simulink model "quadruped"  (R2019b)
settings: Solver=ode23t  StartTime=0.0  StopTime=Ts  RelTol=1e-3
values from neighbouring files (symbols this model uses):
  isdone = Isdone    [RL_reward.m]
  plane = [5, 50, 0.03]    [quadruped_sim_param.m]
  reward = Reward    [RL_reward.m]
  robot = Robot    [quadruped_sim_param.m]
undefined symbols (not defined in the file or in its folder): X, Y, Z
libraries: sm_lib x166, nesl_utility x90, simulink x33, rllib x1
(part 1 of 6)
settings Model: Creator=krzysiek  LastModifiedBy=dimazhylko
settings SolverCC: ZeroCrossAlgorithm=Adaptive
settings DebuggingCC: IgnoredZcDiagnostic=none
settings DiagnosticsConfigSet: SimMechanicsRigidlyBoundBlock=none

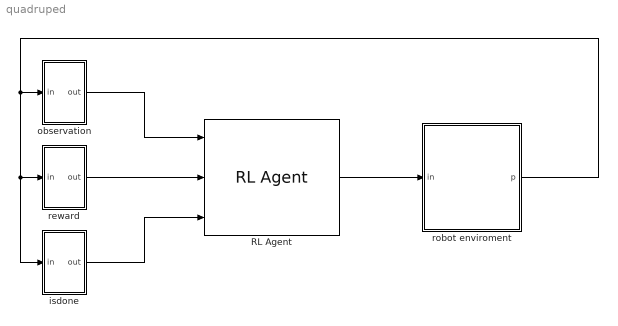
== system quadruped ==
  RL Agent : rllib/RL Agent  Agent=agentObj  ProvideReward=on  ProvideIsDone=on  ProvideCumRwd=off  TreatAsDirectFeedthrough=on  CollectLoggedSignals=on  CollectModelStates=on
      settings: SourceProductName=Reinforcement Learning Toolbox
  isdone : Subsystem  mask{isd=isdone}
  observation : Subsystem
  reward : Subsystem  mask{rew=reward}
  robot enviroment : Subsystem
  wires:
  RL Agent/1 -> robot enviroment/1(in)
  robot enviroment/1(p) -> isdone/1(in), reward/1(in), observation/1(in)
  reward/1(out) -> RL Agent/2
  observation/1(out) -> RL Agent/1
  isdone/1(out) -> RL Agent/3

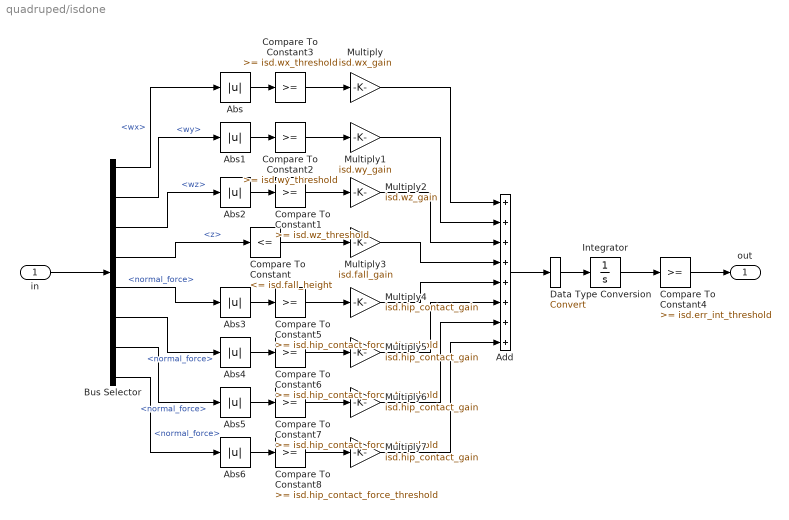
== system quadruped/isdone ==
  in : Inport
  Abs{,1..6} (7 alike) : Abs
  Add : Sum  Inputs=++++++++
  Bus Selector : BusSelector  OutputSignals=body.wx,body.wy,body.wz,body.z,RL.hip.normal_force,FL.hip.normal_force,FR.hip.normal_force,RR.hip.normal_force
  Compare To Constant : simulink/Logic and Bit Operations/Compare To Constant  relop=<=  const=isd.fall_height  OutDataTypeStr=uint8
  Compare To Constant1 : simulink/Logic and Bit Operations/Compare To Constant  relop=>=  const=isd.wz_threshold  OutDataTypeStr=uint8
  Compare To Constant2 : simulink/Logic and Bit Operations/Compare To Constant  relop=>=  const=isd.wy_threshold  OutDataTypeStr=uint8
  Compare To Constant3 : simulink/Logic and Bit Operations/Compare To Constant  relop=>=  const=isd.wx_threshold  OutDataTypeStr=uint8
  Compare To Constant4 : simulink/Logic and Bit Operations/Compare To Constant  relop=>=  const=isd.err_int_threshold  OutDataTypeStr=boolean
  Compare To Constant{5..8} (4 alike) : simulink/Logic and Bit Operations/Compare To Constant  relop=>=  const=isd.hip_contact_force_threshold  OutDataTypeStr=uint8
  Data Type Conversion : DataTypeConversion
  Integrator : Integrator
  Multiply : Gain  Gain=isd.wx_gain
  Multiply1 : Gain  Gain=isd.wy_gain
  Multiply2 : Gain  Gain=isd.wz_gain
  Multiply3 : Gain  Gain=isd.fall_gain
  Multiply{4..7} (4 alike) : Gain  Gain=isd.hip_contact_gain
  out : Outport
  wires:
  in/1 -> Bus Selector/1
  Bus Selector/4 -> Compare To Constant/1  "<z>"
  Abs/1 -> Compare To Constant3/1
  Abs1/1 -> Compare To Constant2/1
  Abs2/1 -> Compare To Constant1/1
  Bus Selector/3 -> Abs2/1  "<wz>"
  Bus Selector/2 -> Abs1/1  "<wy>"
  Bus Selector/1 -> Abs/1  "<wx>"
  Integrator/1 -> Compare To Constant4/1
  Add/1 -> Data Type Conversion/1
  Multiply/1 -> Add/1
  Multiply1/1 -> Add/2
  Multiply2/1 -> Add/3
  Multiply3/1 -> Add/4
  Compare To Constant3/1 -> Multiply/1
  Compare To Constant2/1 -> Multiply1/1
  Compare To Constant1/1 -> Multiply2/1
  Compare To Constant/1 -> Multiply3/1
  Compare To Constant4/1 -> out/1
  Data Type Conversion/1 -> Integrator/1
  Abs3/1 -> Compare To Constant5/1
  Compare To Constant5/1 -> Multiply4/1
  Abs4/1 -> Compare To Constant6/1
  Compare To Constant6/1 -> Multiply5/1
  Abs5/1 -> Compare To Constant7/1
  Compare To Constant7/1 -> Multiply6/1
  Abs6/1 -> Compare To Constant8/1
  Compare To Constant8/1 -> Multiply7/1
  Bus Selector/5 -> Abs3/1  "<normal_force>"
  Bus Selector/6 -> Abs4/1  "<normal_force>"
  Bus Selector/7 -> Abs5/1  "<normal_force>"
  Bus Selector/8 -> Abs6/1  "<normal_force>"
  Multiply5/1 -> Add/6
  Multiply4/1 -> Add/5
  Multiply6/1 -> Add/7
  Multiply7/1 -> Add/8

== system quadruped/observation ==
  in : Inport
  Bus Selector : BusSelector  OutputSignals=RL,FL,FR,RR,body
  Bus Selector{1..4} (4 alike) : BusSelector  OutputSignals=hip.joint.position,leg.lower joint data.position,leg.upper jount data.position,leg.tip.pos,leg.tip.normal_force
  Bus Selector5 : BusSelector  OutputSignals=wx,wy,wz,x,y,z,vx,vy,vz
  Bus Selector{6..9} (4 alike) : BusSelector  OutputSignals=x,y,z
  Mux : Mux  Inputs=37
  out : Outport
  wires:
  in/1 -> Bus Selector/1
  Bus Selector/1 -> Bus Selector1/1  "<RL>"
  Mux/1 -> out/1
  Bus Selector/2 -> Bus Selector2/1  "<FL>"
  Bus Selector/3 -> Bus Selector3/1  "<FR>"
  Bus Selector/4 -> Bus Selector4/1  "<RR>"
  Bus Selector/5 -> Bus Selector5/1  "<body>"
  Bus Selector1/1 -> Mux/1  "<position>"
  Bus Selector1/2 -> Mux/2  "<position>"
  Bus Selector1/3 -> Mux/3  "<position>"
  Bus Selector1/5 -> Mux/7  "<normal_force>"
  Bus Selector2/1 -> Mux/8  "<position>"
  Bus Selector2/2 -> Mux/9  "<position>"
  Bus Selector2/3 -> Mux/10  "<position>"
  Bus Selector2/5 -> Mux/14  "<normal_force>"
  Bus Selector3/1 -> Mux/15  "<position>"
  Bus Selector3/2 -> Mux/16  "<position>"
  Bus Selector3/3 -> Mux/17  "<position>"
  Bus Selector3/5 -> Mux/21  "<normal_force>"
  Bus Selector4/1 -> Mux/22  "<position>"
  Bus Selector4/2 -> Mux/23  "<position>"
  Bus Selector4/3 -> Mux/24  "<position>"
  Bus Selector5/2 -> Mux/30  "<wy>"
  Bus Selector5/3 -> Mux/31  "<wz>"
  Bus Selector5/4 -> Mux/32  "<x>"
  Bus Selector5/5 -> Mux/33  "<y>"
  Bus Selector5/6 -> Mux/34  "<z>"
  Bus Selector5/7 -> Mux/35  "<vx>"
  Bus Selector5/8 -> Mux/36  "<vy>"
  Bus Selector5/9 -> Mux/37  "<vz>"
  Bus Selector2/4 -> Bus Selector6/1  "<pos>"
  Bus Selector6/1 -> Mux/11  "<x>"
  Bus Selector6/2 -> Mux/12  "<y>"
  Bus Selector6/3 -> Mux/13  "<z>"
  Bus Selector1/4 -> Bus Selector7/1  "<pos>"
  Bus Selector7/1 -> Mux/4  "<x>"
  Bus Selector7/2 -> Mux/5  "<y>"
  Bus Selector7/3 -> Mux/6  "<z>"
  Bus Selector4/4 -> Bus Selector8/1  "<pos>"
  Bus Selector8/1 -> Mux/25  "<x>"
  Bus Selector5/1 -> Mux/29  "<wx>"
  Bus Selector8/2 -> Mux/26  "<y>"
  Bus Selector8/3 -> Mux/27  "<z>"
  Bus Selector4/5 -> Mux/28  "<normal_force>"
  Bus Selector3/4 -> Bus Selector9/1  "<pos>"
  Bus Selector9/1 -> Mux/18  "<x>"
  Bus Selector9/2 -> Mux/19  "<y>"
  Bus Selector9/3 -> Mux/20  "<z>"

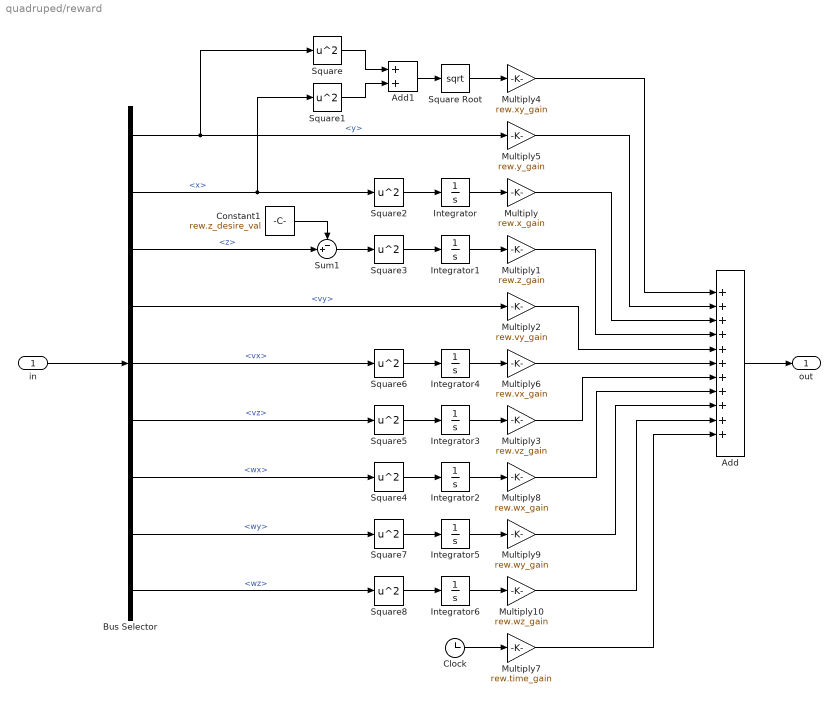
== system quadruped/reward ==
  in : Inport
  Add : Sum  Inputs=+++++++++++
  Add1 : Sum
  Bus Selector : BusSelector  OutputSignals=body.y,body.x,body.z,body.vy,body.vx,body.vz,body.wx,body.wy,body.wz
  Clock : Clock
  Constant1 : Constant  Value=rew.z_desire_val
  Integrator{,1..6} (7 alike) : Integrator
  Multiply : Gain  Gain=rew.x_gain
  Multiply1 : Gain  Gain=rew.z_gain
  Multiply10 : Gain  Gain=rew.wz_gain
  Multiply2 : Gain  Gain=rew.vy_gain
  Multiply3 : Gain  Gain=rew.vz_gain
  Multiply4 : Gain  Gain=rew.xy_gain
  Multiply5 : Gain  Gain=rew.y_gain
  Multiply6 : Gain  Gain=rew.vx_gain
  Multiply7 : Gain  Gain=rew.time_gain
  Multiply8 : Gain  Gain=rew.wx_gain
  Multiply9 : Gain  Gain=rew.wy_gain
  Square : Math  Operator=square  RndMeth=Zero  SaturateOnIntegerOverflow=on
  Square Root : Sqrt  SaturateOnIntegerOverflow=on
  Square1 : Math  Operator=square  RndMeth=Zero  SaturateOnIntegerOverflow=on
  Square{2..8} (7 alike) : Math  Operator=square  SignedPower=off  SaturateOnIntegerOverflow=on
  Sum1 : Sum  Inputs=-+|
  out : Outport
  wires:
  in/1 -> Bus Selector/1
  Square2/1 -> Integrator/1
  Square3/1 -> Integrator1/1
  Sum1/1 -> Square3/1
  Constant1/1 -> Sum1/1
  Square5/1 -> Integrator3/1
  Integrator/1 -> Multiply/1
  Integrator3/1 -> Multiply3/1
  Integrator1/1 -> Multiply1/1
  Add/1 -> out/1
  Add1/1 -> Square Root/1
  Square/1 -> Add1/1
  Square1/1 -> Add1/2
  Square Root/1 -> Multiply4/1
  Multiply4/1 -> Add/1
  Multiply5/1 -> Add/2
  Multiply/1 -> Add/3
  Multiply1/1 -> Add/4
  Multiply6/1 -> Add/6
  Clock/1 -> Multiply7/1
  Multiply3/1 -> Add/7
  Square6/1 -> Integrator4/1
  Integrator4/1 -> Multiply6/1
  Multiply2/1 -> Add/5
  Bus Selector/1 -> Multiply5/1, Square/1  "<y>"
  Bus Selector/2 -> Square2/1, Square1/1  "<x>"
  Bus Selector/3 -> Sum1/2  "<z>"
  Bus Selector/4 -> Multiply2/1  "<vy>"
  Bus Selector/5 -> Square6/1  "<vx>"
  Bus Selector/6 -> Square5/1  "<vz>"
  Square4/1 -> Integrator2/1
  Integrator2/1 -> Multiply8/1
  Square7/1 -> Integrator5/1
  Integrator5/1 -> Multiply9/1
  Square8/1 -> Integrator6/1
  Integrator6/1 -> Multiply10/1
  Bus Selector/7 -> Square4/1  "<wx>"
  Bus Selector/8 -> Square7/1  "<wy>"
  Bus Selector/9 -> Square8/1  "<wz>"
  Multiply8/1 -> Add/8
  Multiply9/1 -> Add/9
  Multiply10/1 -> Add/10
  Multiply7/1 -> Add/11

== system quadruped/robot enviroment ==
  in : Inport
  Bus Creator : BusCreator  Inputs=5
  FL : Subsystem  mask{Leg=robot.RL, plane_dim=plane}
  FR : Subsystem  mask{Leg=robot.FR, plane_dim=plane}
  Mechanism Configuration : sm_lib/Utilities/Mechanism Configuration  UniformGravity=Constant  GravityVector=[0 0 -9.80665]  GravityUnits=m/s^2  LinearizationDelta=0.001
  "Plane " : sm_lib/Body Elements/Brick Solid  GraphicAmbientColor=[0.15 0.15 0.15 1.0]  BasedOnType=Density  BrickDimensions=plane  BrickDimensionUnits=m  CenterOfMass=[0 0 0]  CenterOfMassUnits=m  GraphicDiffuseColor=[0.5 0.5 0.5]  Density=1000  DensityUnits=kg/m^3  DoExposeReferenceFrame=on  GraphicEmissiveColor=[0.0 0.0 0.0 1.0]  ExportEntireGeometry=on  SerializedFrames=<Frames/>  MarkerShape=Sphere  MarkerSize=10  GraphicType=FromGeometry  InertiaType=CalculateFromGeometry  Mass=1  MassUnits=kg  MomentsOfInertia=[1 1 1]  MomentsOfInertiaUnits=kg*m^2  GraphicOpacity=1.0  ProductsOfInertia=[0 0 0]  ProductsOfInertiaUnits=kg*m^2  GraphicShininess=75  GraphicSpecularColor=[0.5 0.5 0.5 1.0]  GraphicVisPropType=SimpleVisualProperties
  RL : Subsystem  mask{Leg=robot.RL, plane_dim=plane}
  RR : Subsystem  mask{Leg=robot.RR, plane_dim=plane}
  Solver Configuration : nesl_utility/Solver Configuration  PhysicalDomain=network_engine_domain  SubClassName=solver  LeftPortType=input  RightPortType=generic  Tones=[]  Harmonics=[]  SimulateNoise=off  Profile=off  UseLocalSampling=off  EnableSwitchedLinearOptims=on  FrequencyDomain=off  UseCCode=off  RelTol=0.001  AbsTol=1e-06  MinStep=1e-09  ToWorkspace=off  RevertToSquareIcSolve=off  NumHomotopyIterations=100  PhasorMode=off  PhasorModeNumHarmonics=1  DoDC=off  ResidualTolerance=1e-09  UseLocalSolver=off  LocalSolverChoice=NE_TRAPEZOIDAL_ADVANCER  LocalSolverSampleTime=0.1  DoFixedCost=off  MaxNonlinIter=3  MaxModeIter=2  LinearAlgebra=Sparse  EquationFormulation=NE_TIME_EF  DelaysMemoryBudget=1024  AutomaticFiltering=on  FilteringTimeConstant=0.001  PartitionStorageMethod=AS_NEEDED  PartitionMemoryBudget=1024  PartitionMethod=FAST
  World Frame : sm_lib/Frames and Transforms/World Frame
  fancy data manipulation : Subsystem
  robot body : Subsystem  mask{robot=robot}
  p : Outport
  wires:
  Bus Creator/1 -> p/1
  robot body/1(p) -> Bus Creator/5  "body"
  RR/1(p) -> Bus Creator/4  "RR"
  FR/1(p) -> Bus Creator/3  "FR"
  FL/1(p) -> Bus Creator/2  "FL"
  RL/1(p) -> Bus Creator/1  "RL"
  in/1 -> fancy data manipulation/1(In1)
  fancy data manipulation/1(Out1) -> RL/1(pos)
  fancy data manipulation/2(Out2) -> FL/1(pos)
  fancy data manipulation/3(Out3) -> RR/1(pos)
  fancy data manipulation/4(Out4) -> FR/1(pos)
  connections:
  RL/RConn2 -- FL/RConn2 -- FR/RConn2 -- RR/RConn2 -- "Plane "/RConn1 -- robot body/LConn2 -- Solver Configuration/RConn1 -- World Frame/RConn1 -- Mechanism Configuration/RConn1
  RR/LConn1 -- robot body/LConn3
  robot body/LConn1 -- RL/LConn1
  FL/LConn1 -- robot body/RConn1
  FR/LConn1 -- robot body/RConn2
  RL/RConn1 -- FL/RConn1 -- FR/RConn1 -- RR/RConn1 -- "Plane "/LConn1

== system quadruped/robot enviroment/FL ==
  pos : Inport
  Bus Creator : BusCreator  Inputs=2
  Constant : Constant  Value=90
  Demux : Demux  Outputs=3
  Multiply : Gain  Gain=180/pi
  Sum : Sum  Inputs=|++
  hip : Subsystem  mask{Hip=Leg.hip}
  leg : Subsystem
  plane : PMIOPort  Side=Right
  B : PMIOPort  Port=2  Side=Left
  F : PMIOPort  Port=3  Side=Right
  p : Outport
  wires:
  Demux/3 -> Multiply/1  "hip pos"
  leg/1(p) -> Bus Creator/2  "leg"
  Bus Creator/1 -> p/1
  pos/1 -> Demux/1
  Demux/1 -> leg/1(up pos)  "leg ang"
  Demux/2 -> leg/2(lo pos)  "knee ang"
  hip/1(p) -> Bus Creator/1  "hip"
  Multiply/1 -> Sum/1
  Sum/1 -> hip/1(pos)
  Constant/1 -> Sum/2
  connections:
  leg/LConn1 -- hip/RConn1
  hip/LConn1 -- B/RConn1
  hip/RConn2 -- plane/RConn1 -- leg/RConn2
  F/RConn1 -- leg/RConn1

== system quadruped/robot enviroment/FR ==
  pos : Inport
  Bus Creator : BusCreator  Inputs=2
  Constant : Constant  Value=90
  Demux : Demux  Outputs=3
  Multiply : Gain  Gain=180/pi
  Sum : Sum  Inputs=|++
  hip : Subsystem  mask{Hip=Leg.hip}
  leg : Subsystem
  plane : PMIOPort  Side=Right
  B : PMIOPort  Port=2  Side=Left
  F : PMIOPort  Port=3  Side=Right
  p : Outport
  wires:
  Demux/3 -> Multiply/1  "hip pos"
  leg/1(p) -> Bus Creator/2  "leg"
  Bus Creator/1 -> p/1
  pos/1 -> Demux/1
  Demux/1 -> leg/1(up pos)  "leg ang"
  Demux/2 -> leg/2(lo pos)  "knee ang"
  hip/1(p) -> Bus Creator/1  "hip"
  Multiply/1 -> Sum/1
  Sum/1 -> hip/1(pos)
  Constant/1 -> Sum/2
  connections:
  leg/LConn1 -- hip/RConn1
  hip/LConn1 -- B/RConn1
  hip/RConn2 -- plane/RConn1 -- leg/RConn2
  F/RConn1 -- leg/RConn1

== system quadruped/robot enviroment/RL ==
  pos : Inport
  Bus Creator : BusCreator  Inputs=2
  Constant : Constant  Value=90
  Demux : Demux  Outputs=3
  Multiply : Gain  Gain=180/pi
  Sum : Sum  Inputs=|++
  hip : Subsystem  mask{Hip=Leg.hip}
  leg : Subsystem
  plane : PMIOPort  Side=Right
  B : PMIOPort  Port=2  Side=Left
  F : PMIOPort  Port=3  Side=Right
  p : Outport
  wires:
  Demux/3 -> Multiply/1  "hip pos"
  leg/1(p) -> Bus Creator/2  "leg"
  Bus Creator/1 -> p/1
  pos/1 -> Demux/1
  Demux/1 -> leg/1(up pos)  "leg ang"
  Demux/2 -> leg/2(lo pos)  "knee ang"
  hip/1(p) -> Bus Creator/1  "hip"
  Multiply/1 -> Sum/1
  Sum/1 -> hip/1(pos)
  Constant/1 -> Sum/2
  connections:
  leg/LConn1 -- hip/RConn1
  hip/LConn1 -- B/RConn1
  hip/RConn2 -- plane/RConn1 -- leg/RConn2
  F/RConn1 -- leg/RConn1

== system quadruped/robot enviroment/RR ==
  pos : Inport
  Bus Creator : BusCreator  Inputs=2
  Constant : Constant  Value=90
  Demux : Demux  Outputs=3
  Multiply : Gain  Gain=180/pi
  Sum : Sum  Inputs=|++
  hip : Subsystem  mask{Hip=Leg.hip}
  leg : Subsystem
  plane : PMIOPort  Side=Right
  B : PMIOPort  Port=2  Side=Left
  F : PMIOPort  Port=3  Side=Right
  p : Outport
  wires:
  Demux/3 -> Multiply/1  "hip pos"
  leg/1(p) -> Bus Creator/2  "leg"
  Bus Creator/1 -> p/1
  pos/1 -> Demux/1
  Demux/1 -> leg/1(up pos)  "leg ang"
  Demux/2 -> leg/2(lo pos)  "knee ang"
  hip/1(p) -> Bus Creator/1  "hip"
  Multiply/1 -> Sum/1
  Sum/1 -> hip/1(pos)
  Constant/1 -> Sum/2
  connections:
  leg/LConn1 -- hip/RConn1
  hip/LConn1 -- B/RConn1
  hip/RConn2 -- plane/RConn1 -- leg/RConn2
  F/RConn1 -- leg/RConn1

== system quadruped/robot enviroment/fancy data manipulation ==
  In1 : Inport
  Demux : Demux  Outputs=12
  Mux{,1..3} (4 alike) : Mux  Inputs=3
  Out1 : Outport
  Out2 : Outport  Port=2
  Out3 : Outport  Port=3
  Out4 : Outport  Port=4
  wires:
  Mux/1 -> Out1/1
  Mux1/1 -> Out2/1
  Mux3/1 -> Out3/1
  In1/1 -> Demux/1
  Mux2/1 -> Out4/1
  Demux/1 -> Mux/1
  Demux/2 -> Mux1/1
  Demux/3 -> Mux2/1
  Demux/4 -> Mux3/1
  Demux/5 -> Mux/2
  Demux/6 -> Mux1/2
  Demux/7 -> Mux2/2
  Demux/8 -> Mux3/2
  Demux/9 -> Mux/3
  Demux/10 -> Mux1/3
  Demux/11 -> Mux2/3
  Demux/12 -> Mux3/3

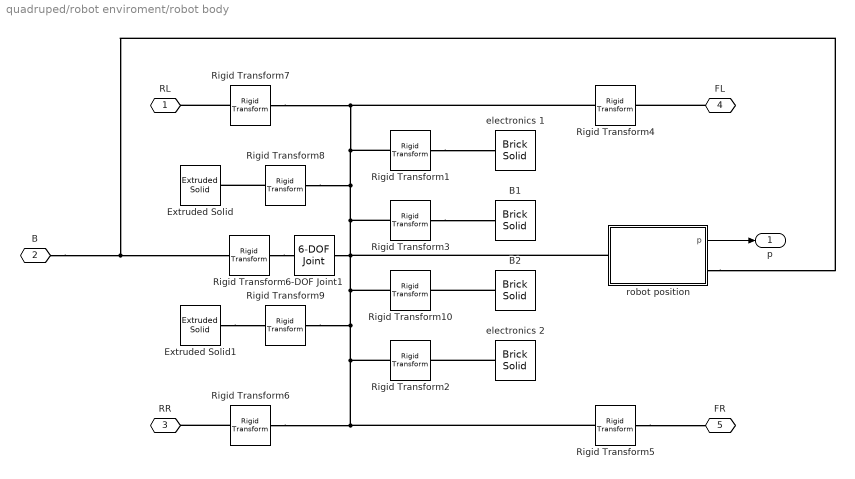
== system quadruped/robot enviroment/robot body ==
  6-DOF Joint1 : sm_lib/Joints/6-DOF Joint  JointMode=Normal  SenseConstraintForce=off  SenseConstraintForceX=off  SenseConstraintForceY=off  SenseConstraintForceZ=off  SenseConstraintTorque=off  SenseConstraintTorqueX=off  SenseConstraintTorqueY=off  SenseConstraintTorqueZ=off  SenseTotalForce=off  SenseTotalForceX=off  SenseTotalForceY=off  SenseTotalForceZ=off  SenseTotalTorque=off  SenseTotalTorqueX=off  SenseTotalTorqueY=off  SenseTotalTorqueZ=off  CompositeWrenchDir=FollowerOnBase  CompositeWrenchFrame=BaseFrame  PxEquilibriumPosition=0  PxEquilibriumPositionUnits=m  PxSpringStiffness=0  PxSpringStiffnessUnits=N/m  PxDampingCoefficient=0  PxDampingCoefficientUnits=N/(m/s)  PxTorqueActuationMode=NoTorque  PxMotionActuationMode=ComputedMotion  PxSensePosition=off  PxSenseVelocity=off  PxSenseAcceleration=off  PxSenseTorqueForce=off  PxSenseLowerLimitTorqueForce=off  PxSenseUpperLimitTorqueForce=off  PxLowerLimitSpecify=off  PxLowerLimitBound=-1  PxLowerLimitBoundUnits=m  PxLowerLimitStiffness=1e6  PxLowerLimitStiffnessUnits=N/m  PxLowerLimitDamping=1e3  PxLowerLimitDampingUnits=N/(m/s)  PxLowerLimitTransitionRegionWidth=1e-4  PxLowerLimitTransitionRegionWidthUnits=m  PxUpperLimitSpecify=off  PxUpperLimitBound=1  PxUpperLimitBoundUnits=m  PxUpperLimitStiffness=1e6  PxUpperLimitStiffnessUnits=N/m  PxUpperLimitDamping=1e3  PxUpperLimitDampingUnits=N/(m/s)  PxUpperLimitTransitionRegionWidth=1e-4  PxUpperLimitTransitionRegionWidthUnits=m  PxPositionTargetSpecify=off  PxPositionTargetPriority=High  PxPositionTargetValue=0  PxPositionTargetValueUnits=m  PxVelocityTargetSpecify=off  PxVelocityTargetPriority=High  PxVelocityTargetValue=0  PxVelocityTargetValueUnits=m/s  PyEquilibriumPosition=0  PyEquilibriumPositionUnits=m  PySpringStiffness=0  PySpringStiffnessUnits=N/m  PyDampingCoefficient=0  PyDampingCoefficientUnits=N/(m/s)  PyTorqueActuationMode=NoTorque  PyMotionActuationMode=ComputedMotion  PySensePosition=off  PySenseVelocity=off  PySenseAcceleration=off  PySenseTorqueForce=off  PySenseLowerLimitTorqueForce=off  PySenseUpperLimitTorqueForce=off  PyLowerLimitSpecify=off  PyLowerLimitBound=-1  PyLowerLimitBoundUnits=m  PyLowerLimitStiffness=1e6  PyLowerLimitStiffnessUnits=N/m  PyLowerLimitDamping=1e3  PyLowerLimitDampingUnits=N/(m/s)  PyLowerLimitTransitionRegionWidth=1e-4  PyLowerLimitTransitionRegionWidthUnits=m  PyUpperLimitSpecify=off  PyUpperLimitBound=1  PyUpperLimitBoundUnits=m  PyUpperLimitStiffness=1e6  PyUpperLimitStiffnessUnits=N/m  PyUpperLimitDamping=1e3  PyUpperLimitDampingUnits=N/(m/s)  PyUpperLimitTransitionRegionWidth=1e-4  PyUpperLimitTransitionRegionWidthUnits=m  PyPositionTargetSpecify=off  PyPositionTargetPriority=High  PyPositionTargetValue=0  PyPositionTargetValueUnits=m  PyVelocityTargetSpecify=off  PyVelocityTargetPriority=High  PyVelocityTargetValue=0  PyVelocityTargetValueUnits=m/s  PzEquilibriumPosition=0  PzEquilibriumPositionUnits=m  PzSpringStiffness=0  PzSpringStiffnessUnits=N/m  PzDampingCoefficient=0  PzDampingCoefficientUnits=N/(m/s)  PzTorqueActuationMode=NoTorque  PzMotionActuationMode=ComputedMotion  PzSensePosition=off  PzSenseVelocity=off  PzSenseAcceleration=off  PzSenseTorqueForce=off  PzSenseLowerLimitTorqueForce=off  PzSenseUpperLimitTorqueForce=off  PzLowerLimitSpecify=off  PzLowerLimitBound=-1  PzLowerLimitBoundUnits=m  PzLowerLimitStiffness=1e6  PzLowerLimitStiffnessUnits=N/m  PzLowerLimitDamping=1e3  PzLowerLimitDampingUnits=N/(m/s)  PzLowerLimitTransitionRegionWidth=1e-4  PzLowerLimitTransitionRegionWidthUnits=m  PzUpperLimitSpecify=off  PzUpperLimitBound=1  PzUpperLimitBoundUnits=m  PzUpperLimitStiffness=1e6  PzUpperLimitStiffnessUnits=N/m  PzUpperLimitDamping=1e3  PzUpperLimitDampingUnits=N/(m/s)  PzUpperLimitTransitionRegionWidth=1e-4  PzUpperLimitTransitionRegionWidthUnits=m  PzPositionTargetSpecify=off  PzPositionTargetPriority=High  PzPositionTargetValue=0  PzPositionTargetValueUnits=m  PzVelocityTargetSpecify=off  PzVelocityTargetPriority=High  PzVelocityTargetValue=0  PzVelocityTargetValueUnits=m/s  SphDefPosRotationMethod=None  SphDefPosRotationAngleUnits=deg  SphDefPosRotationStandardAxis=+Z  SphDefPosRotationAngle=0.0  SphDefPosRotationArbitraryAxis=[0 0 1]  SphDefPosFollAlignAxisA=+X  SphDefPosBaseAlignAxisA=+Y  SphDefPosFollAlignAxisB=+Y  SphDefPosBaseAlignAxisB=+Z  SphDefPosRotationSequenceAxes=FollowerAxes  SphDefPosRotationSequence=XYX  SphDefPosRotationSequenceAngles=[0 0 0]  SphDefPosRotationSequenceAnglesUnits=deg  SphDefPosRotationMatrix=[1 0 0; 0 1 0; 0 0 1]  SphEqPosRotationMethod=None  SphEqPosRotationAngleUnits=deg  SphEqPosRotationStandardAxis=+Z  SphEqPosRotationAngle=0.0  SphEqPosRotationArbitraryAxis=[0 0 1]  SphEqPosFollAlignAxisA=+X  SphEqPosBaseAlignAxisA=+Y  SphEqPosFollAlignAxisB=+Y  SphEqPosBaseAlignAxisB=+Z  SphEqPosRotationSequenceAxes=FollowerAxes  SphEqPosRotationSequence=XYX  SphEqPosRotationSequenceAngles=[0 0 0]  SphEqPosRotationSequenceAnglesUnits=deg  SphEqPosRotationMatrix=[1 0 0; 0 1 0; 0 0 1]  SphSpringStiffness=0  SphSpringStiffnessUnits=N*m/deg  SphDampingCoefficient=0  SphDampingCoefficientUnits=N*m/(deg/s)  SphActuateTorqueX=off  SphActuateTorqueY=off  SphActuateTorqueZ=off  SphActuateTorque=off  SphTorqueActuationMode=NoTorque  SphMotionActuationMode=ComputedMotion  SphActuationFrame=BaseFrame  SphSensePosition=off  SphSenseVelocityX=off  SphSenseVelocityY=off  SphSenseVelocityZ=off  SphSenseVelocity=off  SphSenseAccelerationX=off  SphSenseAccelerationY=off  SphSenseAccelerationZ=off  SphSenseAcceleration=off  SphSenseTorqueX=off  SphSenseTorqueY=off  SphSenseTorqueZ=off  SphSenseTorqueForce=off  SphSenseLowerLimitTorqueMag=off  SphSenseUpperLimitTorqueMag=off  SphSensingFrame=BaseFrame  SphLowerLimitSpecify=off  SphLowerLimitBound=15  SphLowerLimitBoundUnits=deg  SphLowerLimitStiffness=1e4  SphLowerLimitStiffnessUnits=N*m/deg  SphLowerLimitDamping=10  SphLowerLimitDampingUnits=N*m/(deg/s)  SphLowerLimitTransitionRegionWidth=0.1  SphLowerLimitTransitionRegionWidthUnits=deg  SphUpperLimitSpecify=off  SphUpperLimitBound=45  SphUpperLimitBoundUnits=deg  SphUpperLimitStiffness=1e4  SphUpperLimitStiffnessUnits=N*m/deg  SphUpperLimitDamping=10  SphUpperLimitDampingUnits=N*m/(deg/s)  SphUpperLimitTransitionRegionWidth=0.1  SphUpperLimitTransitionRegionWidthUnits=deg  SphPositionTargetRotationMethod=None  SphPositionTargetRotationAngleUnits=deg  SphPositionTargetRotationStandardAxis=+Z  SphPositionTargetRotationAngle=0.0  SphPositionTargetRotationArbitraryAxis=[0 0 1]  SphPositionTargetFollAlignAxisA=+X  SphPositionTargetBaseAlignAxisA=+Y  SphPositionTargetFollAlignAxisB=+Y  SphPositionTargetBaseAlignAxisB=+Z  SphPositionTargetRotationSequenceAxes=FollowerAxes  SphPositionTargetRotationSequence=XYX  SphPositionTargetRotationSequenceAngles=[0 0 0]  SphPositionTargetRotationSequenceAnglesUnits=deg  SphPositionTargetRotationMatrix=[1 0 0; 0 1 0; 0 0 1]  SphPositionTargetSpecify=off  SphPositionTargetPriority=High  SphVelocityTargetValue=[0 0 0]  SphVelocityTargetValueUnits=deg/s  SphVelocityTargetSpecify=off  SphVelocityTargetPriority=High  SphVelocityTargetInFollowerFrame=on
  B1 : sm_lib/Body Elements/Brick Solid  GraphicAmbientColor=[0.15 0.15 0.15 1.0]  BasedOnType=Mass  BrickDimensions=robot.b1.dimension  BrickDimensionUnits=mm  CenterOfMass=[0 0 0]  CenterOfMassUnits=m  GraphicDiffuseColor=robot.b1.color  Density=robot.b1.density  DensityUnits=kg/m^3  DoExposeReferenceFrame=on  GraphicEmissiveColor=[0.0 0.0 0.0 1.0]  ExportEntireGeometry=off  SerializedFrames=<Frames/>  MarkerShape=Sphere  MarkerSize=10  GraphicType=FromGeometry  InertiaType=CalculateFromGeometry  Mass=robot.b1.mass  MassUnits=g  MomentsOfInertia=[1 1 1]  MomentsOfInertiaUnits=kg*m^2  GraphicOpacity=1.0  ProductsOfInertia=[0 0 0]  ProductsOfInertiaUnits=kg*m^2  GraphicShininess=75  GraphicSpecularColor=[0.5 0.5 0.5 1.0]  GraphicVisPropType=SimpleVisualProperties
  B2 : sm_lib/Body Elements/Brick Solid  GraphicAmbientColor=[0.15 0.15 0.15 1.0]  BasedOnType=Mass  BrickDimensions=robot.b2.dimension  BrickDimensionUnits=mm  CenterOfMass=[0 0 0]  CenterOfMassUnits=m  GraphicDiffuseColor=robot.b1.color  Density=robot.b2.density  DensityUnits=kg/m^3  DoExposeReferenceFrame=on  GraphicEmissiveColor=[0.0 0.0 0.0 1.0]  ExportEntireGeometry=off  SerializedFrames=<Frames/>  MarkerShape=Sphere  MarkerSize=10  GraphicType=FromGeometry  InertiaType=CalculateFromGeometry  Mass=robot.b1.mass  MassUnits=g  MomentsOfInertia=[1 1 1]  MomentsOfInertiaUnits=kg*m^2  GraphicOpacity=1.0  ProductsOfInertia=[0 0 0]  ProductsOfInertiaUnits=kg*m^2  GraphicShininess=75  GraphicSpecularColor=[0.5 0.5 0.5 1.0]  GraphicVisPropType=SimpleVisualProperties
  Extruded Solid : sm_lib/Body Elements/Extruded Solid  GraphicAmbientColor=[0.15 0.15 0.15 1.0]  BasedOnType=Mass  CenterOfMass=[0 0 0]  CenterOfMassUnits=m  GraphicDiffuseColor=robot.enclosure.color  ExtrusionCrossSection=[1 1; -1 1; -1 -1; 1 -1]  ExtrusionCrossSectionUnits=m  Density=robot.enclosure.density  DensityUnits=kg/m^3  DoExposeReferenceFrame=on  GraphicEmissiveColor=[0.0 0.0 0.0 1.0]  ExportEntireGeometry=off  ExtrusionLength=robot.enclosure.dimension(3)  ExtrusionLengthUnits=mm  ExtrusionType=Regular  SerializedFrames=<Frames/>  MarkerShape=Sphere  MarkerSize=10  GraphicType=FromGeometry  InertiaType=CalculateFromGeometry  Mass=robot.enclosure.mass  MassUnits=g  MomentsOfInertia=[1 1 1]  MomentsOfInertiaUnits=kg*m^2  PolygonNumSides=6  GraphicOpacity=robot.enclosure.opacity  PolygonOuterRadius=robot.enclosure.dimension(1)  PolygonOuterRadiusUnits=mm  ProductsOfInertia=[0 0 0]  ProductsOfInertiaUnits=kg*m^2  GraphicShininess=75  GraphicSpecularColor=[0.5 0.5 0.5 1.0]  GraphicVisPropType=SimpleVisualProperties
      settings: SourceProductName=Simscape Multibody
  Extruded Solid1 : sm_lib/Body Elements/Extruded Solid  GraphicAmbientColor=[0.15 0.15 0.15 1.0]  BasedOnType=Mass  CenterOfMass=[0 0 0]  CenterOfMassUnits=m  GraphicDiffuseColor=robot.enclosure.color  ExtrusionCrossSection=[1 1; -1 1; -1 -1; 1 -1]  ExtrusionCrossSectionUnits=m  Density=robot.enclosure.density  DensityUnits=kg/m^3  DoExposeReferenceFrame=on  GraphicEmissiveColor=[0.0 0.0 0.0 1.0]  ExportEntireGeometry=off  ExtrusionLength=robot.enclosure.dimension(3)  ExtrusionLengthUnits=mm  ExtrusionType=Regular  SerializedFrames=<Frames/>  MarkerShape=Sphere  MarkerSize=10  GraphicType=FromGeometry  InertiaType=CalculateFromGeometry  Mass=robot.enclosure.mass  MassUnits=g  MomentsOfInertia=[1 1 1]  MomentsOfInertiaUnits=kg*m^2  PolygonNumSides=6  GraphicOpacity=robot.enclosure.opacity  PolygonOuterRadius=robot.enclosure.dimension(1)  PolygonOuterRadiusUnits=mm  ProductsOfInertia=[0 0 0]  ProductsOfInertiaUnits=kg*m^2  GraphicShininess=75  GraphicSpecularColor=[0.5 0.5 0.5 1.0]  GraphicVisPropType=SimpleVisualProperties
      settings: SourceProductName=Simscape Multibody
  Rigid Transform : sm_lib/Frames and Transforms/Rigid Transform  TranslationMethod=StandardAxis  TranslationStandardOffset=340  TranslationLengthUnit=mm  TranslationStandardAxis=+Z  TranslationCartesianOffset=[0 0 0]  TranslationROffset=0  TranslationROffsetUnits=m  TranslationZOffset=0  TranslationZOffsetUnits=m  TranslationThetaOffset=0  TranslationThetaOffsetUnits=deg  RotationMethod=None  RotationAngleUnits=deg  RotationStandardAxis=+Z  RotationAngle=0.0  RotationArbitraryAxis=[0 0 1]  FollAlignAxisA=+X  BaseAlignAxisA=+Y  FollAlignAxisB=+Y  BaseAlignAxisB=+Z  RotationSequenceAxes=FollowerAxes  RotationSequence=XYX  RotationSequenceAngles=[0 0 0]  RotationSequenceAnglesUnits=deg  RotationMatrix=[1 0 0; 0 1 0; 0 0 1]
  Rigid Transform1 : sm_lib/Frames and Transforms/Rigid Transform  TranslationMethod=Cartesian  TranslationStandardOffset=0  TranslationLengthUnit=mm  TranslationStandardAxis=+Z  TranslationCartesianOffset=robot.odrv_l.position  TranslationROffset=0  TranslationROffsetUnits=m  TranslationZOffset=0  TranslationZOffsetUnits=m  TranslationThetaOffset=0  TranslationThetaOffsetUnits=deg  RotationMethod=StandardAxis  RotationAngleUnits=deg  RotationStandardAxis=+X  RotationAngle=90  RotationArbitraryAxis=[0 0 1]  FollAlignAxisA=+X  BaseAlignAxisA=+Y  FollAlignAxisB=+Y  BaseAlignAxisB=+Z  RotationSequenceAxes=FollowerAxes  RotationSequence=XYX  RotationSequenceAngles=[0 0 0]  RotationSequenceAnglesUnits=deg  RotationMatrix=[1 0 0; 0 1 0; 0 0 1]
  Rigid Transform10 : sm_lib/Frames and Transforms/Rigid Transform  TranslationMethod=Cartesian  TranslationStandardOffset=0  TranslationLengthUnit=mm  TranslationStandardAxis=+Z  TranslationCartesianOffset=robot.b2.position  TranslationROffset=0  TranslationROffsetUnits=m  TranslationZOffset=0  TranslationZOffsetUnits=m  TranslationThetaOffset=0  TranslationThetaOffsetUnits=deg  RotationMethod=StandardAxis  RotationAngleUnits=deg  RotationStandardAxis=+X  RotationAngle=90  RotationArbitraryAxis=[0 0 1]  FollAlignAxisA=+X  BaseAlignAxisA=+Y  FollAlignAxisB=+Y  BaseAlignAxisB=+Z  RotationSequenceAxes=FollowerAxes  RotationSequence=XYX  RotationSequenceAngles=[0 0 0]  RotationSequenceAnglesUnits=deg  RotationMatrix=[1 0 0; 0 1 0; 0 0 1]
  Rigid Transform2 : sm_lib/Frames and Transforms/Rigid Transform  TranslationMethod=Cartesian  TranslationStandardOffset=0  TranslationLengthUnit=mm  TranslationStandardAxis=+Z  TranslationCartesianOffset=robot.odrv_r.position  TranslationROffset=0  TranslationROffsetUnits=m  TranslationZOffset=0  TranslationZOffsetUnits=m  TranslationThetaOffset=0  TranslationThetaOffsetUnits=deg  RotationMethod=StandardAxis  RotationAngleUnits=deg  RotationStandardAxis=+X  RotationAngle=90  RotationArbitraryAxis=[0 0 1]  FollAlignAxisA=+X  BaseAlignAxisA=+Y  FollAlignAxisB=+Y  BaseAlignAxisB=+Z  RotationSequenceAxes=FollowerAxes  RotationSequence=XYX  RotationSequenceAngles=[0 0 0]  RotationSequenceAnglesUnits=deg  RotationMatrix=[1 0 0; 0 1 0; 0 0 1]
  Rigid Transform3 : sm_lib/Frames and Transforms/Rigid Transform  TranslationMethod=Cartesian  TranslationStandardOffset=0  TranslationLengthUnit=mm  TranslationStandardAxis=+Z  TranslationCartesianOffset=robot.b1.position  TranslationROffset=0  TranslationROffsetUnits=m  TranslationZOffset=0  TranslationZOffsetUnits=m  TranslationThetaOffset=0  TranslationThetaOffsetUnits=deg  RotationMethod=StandardAxis  RotationAngleUnits=deg  RotationStandardAxis=+X  RotationAngle=90  RotationArbitraryAxis=[0 0 1]  FollAlignAxisA=+X  BaseAlignAxisA=+Y  FollAlignAxisB=+Y  BaseAlignAxisB=+Z  RotationSequenceAxes=FollowerAxes  RotationSequence=XYX  RotationSequenceAngles=[0 0 0]  RotationSequenceAnglesUnits=deg  RotationMatrix=[1 0 0; 0 1 0; 0 0 1]
  Rigid Transform4 : sm_lib/Frames and Transforms/Rigid Transform  TranslationMethod=Cartesian  TranslationStandardOffset=0  TranslationLengthUnit=mm  TranslationStandardAxis=+Z  TranslationCartesianOffset=[-robot.body.dimension(1)/2, robot.body.dimension(2)/2, 0]  TranslationROffset=0  TranslationROffsetUnits=m  TranslationZOffset=0  TranslationZOffsetUnits=m  TranslationThetaOffset=0  TranslationThetaOffsetUnits=deg  RotationMethod=RotationSequence  RotationAngleUnits=deg  RotationStandardAxis=+Z  RotationAngle=0.0  RotationArbitraryAxis=[0 0 1]  FollAlignAxisA=+X  BaseAlignAxisA=+Y  FollAlignAxisB=+Y  BaseAlignAxisB=+Z  RotationSequenceAxes=FollowerAxes  RotationSequence=XYZ  RotationSequenceAngles=[-90 0 90]  RotationSequenceAnglesUnits=deg  RotationMatrix=[1 0 0; 0 1 0; 0 0 1]
  Rigid Transform5 : sm_lib/Frames and Transforms/Rigid Transform  TranslationMethod=Cartesian  TranslationStandardOffset=0  TranslationLengthUnit=mm  TranslationStandardAxis=+Z  TranslationCartesianOffset=[robot.body.dimension(1)/2, robot.body.dimension(2)/2, 0]  TranslationROffset=0  TranslationROffsetUnits=m  TranslationZOffset=0  TranslationZOffsetUnits=m  TranslationThetaOffset=0  TranslationThetaOffsetUnits=deg  RotationMethod=RotationSequence  RotationAngleUnits=deg  RotationStandardAxis=+Z  RotationAngle=0.0  RotationArbitraryAxis=[0 0 1]  FollAlignAxisA=+X  BaseAlignAxisA=+Y  FollAlignAxisB=+Y  BaseAlignAxisB=+Z  RotationSequenceAxes=FollowerAxes  RotationSequence=XYZ  RotationSequenceAngles=[-90 0 90]  RotationSequenceAnglesUnits=deg  RotationMatrix=[1 0 0; 0 1 0; 0 0 1]
  Rigid Transform6 : sm_lib/Frames and Transforms/Rigid Transform  TranslationMethod=Cartesian  TranslationStandardOffset=0  TranslationLengthUnit=mm  TranslationStandardAxis=+Z  TranslationCartesianOffset=[robot.body.dimension(1)/2, -robot.body.dimension(2)/2, 0]  TranslationROffset=0  TranslationROffsetUnits=m  TranslationZOffset=0  TranslationZOffsetUnits=m  TranslationThetaOffset=0  TranslationThetaOffsetUnits=deg  RotationMethod=RotationSequence  RotationAngleUnits=deg  RotationStandardAxis=+Z  RotationAngle=90  RotationArbitraryAxis=[0 0 1]  FollAlignAxisA=+X  BaseAlignAxisA=+Y  FollAlignAxisB=+Y  BaseAlignAxisB=+Z  RotationSequenceAxes=FollowerAxes  RotationSequence=XYZ  RotationSequenceAngles=[-90 0 90]  RotationSequenceAnglesUnits=deg  RotationMatrix=[1 0 0; 0 1 0; 0 0 1]
  Rigid Transform7 : sm_lib/Frames and Transforms/Rigid Transform  TranslationMethod=Cartesian  TranslationStandardOffset=0  TranslationLengthUnit=mm  TranslationStandardAxis=+Z  TranslationCartesianOffset=[-robot.body.dimension(1)/2, -robot.body.dimension(2)/2, 0]  TranslationROffset=0  TranslationROffsetUnits=m  TranslationZOffset=0  TranslationZOffsetUnits=m  TranslationThetaOffset=0  TranslationThetaOffsetUnits=deg  RotationMethod=RotationSequence  RotationAngleUnits=deg  RotationStandardAxis=+Z  RotationAngle=0.0  RotationArbitraryAxis=[0 0 1]  FollAlignAxisA=+X  BaseAlignAxisA=+Y  FollAlignAxisB=+Y  BaseAlignAxisB=+Z  RotationSequenceAxes=FollowerAxes  RotationSequence=XYZ  RotationSequenceAngles=[90 180 -90]  RotationSequenceAnglesUnits=deg  RotationMatrix=[1 0 0; 0 1 0; 0 0 1]
  Rigid Transform8 : sm_lib/Frames and Transforms/Rigid Transform  TranslationMethod=Cartesian  TranslationStandardOffset=0  TranslationLengthUnit=mm  TranslationStandardAxis=+Z  TranslationCartesianOffset=robot.enclosure.position  TranslationROffset=0  TranslationROffsetUnits=m  TranslationZOffset=0  TranslationZOffsetUnits=m  TranslationThetaOffset=0  TranslationThetaOffsetUnits=deg  RotationMethod=StandardAxis  RotationAngleUnits=deg  RotationStandardAxis=+X  RotationAngle=90  RotationArbitraryAxis=[0 0 1]  FollAlignAxisA=+X  BaseAlignAxisA=+Y  FollAlignAxisB=+Y  BaseAlignAxisB=+Z  RotationSequenceAxes=FollowerAxes  RotationSequence=XYX  RotationSequenceAngles=[0 0 0]  RotationSequenceAnglesUnits=deg  RotationMatrix=[1 0 0; 0 1 0; 0 0 1]
  Rigid Transform9 : sm_lib/Frames and Transforms/Rigid Transform  TranslationMethod=Cartesian  TranslationStandardOffset=0  TranslationLengthUnit=mm  TranslationStandardAxis=+Z  TranslationCartesianOffset=-robot.enclosure.position  TranslationROffset=0  TranslationROffsetUnits=m  TranslationZOffset=0  TranslationZOffsetUnits=m  TranslationThetaOffset=0  TranslationThetaOffsetUnits=deg  RotationMethod=StandardAxis  RotationAngleUnits=deg  RotationStandardAxis=+X  RotationAngle=90  RotationArbitraryAxis=[0 0 1]  FollAlignAxisA=+X  BaseAlignAxisA=+Y  FollAlignAxisB=+Y  BaseAlignAxisB=+Z  RotationSequenceAxes=FollowerAxes  RotationSequence=XYX  RotationSequenceAngles=[0 0 0]  RotationSequenceAnglesUnits=deg  RotationMatrix=[1 0 0; 0 1 0; 0 0 1]
  electronics 1 : sm_lib/Body Elements/Brick Solid  GraphicAmbientColor=[0.15 0.15 0.15 1.0]  BasedOnType=Mass  BrickDimensions=robot.odrv_l.dimension  BrickDimensionUnits=mm  CenterOfMass=[0 0 0]  CenterOfMassUnits=m  GraphicDiffuseColor=robot.odrv_l.color  Density=1000  DensityUnits=kg/m^3  DoExposeReferenceFrame=on  GraphicEmissiveColor=[0.0 0.0 0.0 1.0]  ExportEntireGeometry=off  SerializedFrames=<Frames/>  MarkerShape=Sphere  MarkerSize=10  GraphicType=FromGeometry  InertiaType=CalculateFromGeometry  Mass=robot.odrv_l.mass  MassUnits=g  MomentsOfInertia=[1 1 1]  MomentsOfInertiaUnits=kg*m^2  GraphicOpacity=1.0  ProductsOfInertia=[0 0 0]  ProductsOfInertiaUnits=kg*m^2  GraphicShininess=75  GraphicSpecularColor=[0.5 0.5 0.5 1.0]  GraphicVisPropType=SimpleVisualProperties
  electronics 2 : sm_lib/Body Elements/Brick Solid  GraphicAmbientColor=[0.15 0.15 0.15 1.0]  BasedOnType=Mass  BrickDimensions=robot.odrv_r.dimension  BrickDimensionUnits=mm  CenterOfMass=[0 0 0]  CenterOfMassUnits=m  GraphicDiffuseColor=robot.odrv_r.color  Density=1000  DensityUnits=kg/m^3  DoExposeReferenceFrame=on  GraphicEmissiveColor=[0.0 0.0 0.0 1.0]  ExportEntireGeometry=off  SerializedFrames=<Frames/>  MarkerShape=Sphere  MarkerSize=10  GraphicType=FromGeometry  InertiaType=CalculateFromGeometry  Mass=robot.odrv_r.mass  MassUnits=g  MomentsOfInertia=[1 1 1]  MomentsOfInertiaUnits=kg*m^2  GraphicOpacity=1.0  ProductsOfInertia=[0 0 0]  ProductsOfInertiaUnits=kg*m^2  GraphicShininess=75  GraphicSpecularColor=[0.5 0.5 0.5 1.0]  GraphicVisPropType=SimpleVisualProperties
  robot position : Subsystem
  RL : PMIOPort  Side=Left
  B : PMIOPort  Port=2  Side=Left
  RR : PMIOPort  Port=3  Side=Left
  FL : PMIOPort  Port=4  Side=Right
  FR : PMIOPort  Port=5  Side=Right
  p : Outport
  wires:
  robot position/1(p) -> p/1
  connections:
  B2/RConn1 -- Rigid Transform10/RConn1
  Rigid Transform3/RConn1 -- B1/RConn1
  Rigid Transform1/RConn1 -- electronics 1/RConn1
  electronics 2/RConn1 -- Rigid Transform2/RConn1
  Rigid Transform3/LConn1 -- 6-DOF Joint1/RConn1 -- robot position/LConn1 -- Rigid Transform10/LConn1 -- Rigid Transform2/LConn1 -- Rigid Transform5/LConn1 -- Rigid Transform6/LConn1 -- Rigid Transform9/LConn1 -- Rigid Transform8/LConn1 -- Rigid Transform1/LConn1 -- Rigid Transform7/LConn1 -- Rigid Transform4/LConn1
  Rigid Transform6/RConn1 -- RR/RConn1
  Rigid Transform7/RConn1 -- RL/RConn1
  FL/RConn1 -- Rigid Transform4/RConn1
  Rigid Transform5/RConn1 -- FR/RConn1
  Rigid Transform8/RConn1 -- Extruded Solid/RConn1
  Extruded Solid1/RConn1 -- Rigid Transform9/RConn1
  B/RConn1 -- robot position/RConn1 -- Rigid Transform/LConn1
  Rigid Transform/RConn1 -- 6-DOF Joint1/LConn1

== system quadruped/robot enviroment/FL/hip ==
  pos : Inport
  Bus Creator : BusCreator  Inputs=2
  PS-Simulink Converter : nesl_utility/PS-Simulink Converter  PhysicalDomain=network_engine_domain  SubClassName=ps_output  LeftPortType=input  RightPortType=output  PseudoPeriodic=off  Frequencies=[]  Unit=N  AffineConversion=off
  Rigid Transform1 : sm_lib/Frames and Transforms/Rigid Transform  TranslationMethod=StandardAxis  TranslationStandardOffset=Hip.gearboxCorrection  TranslationLengthUnit=mm  TranslationStandardAxis=-Z  TranslationCartesianOffset=50  TranslationROffset=0  TranslationROffsetUnits=m  TranslationZOffset=0  TranslationZOffsetUnits=m  TranslationThetaOffset=0  TranslationThetaOffsetUnits=deg  RotationMethod=StandardAxis  RotationAngleUnits=deg  RotationStandardAxis=+Z  RotationAngle=90  RotationArbitraryAxis=[0 0 1]  FollAlignAxisA=+X  BaseAlignAxisA=+Y  FollAlignAxisB=+Y  BaseAlignAxisB=+Z  RotationSequenceAxes=FollowerAxes  RotationSequence=XYZ  RotationSequenceAngles=[180 0 180]  RotationSequenceAnglesUnits=deg  RotationMatrix=[1 0 0; 0 1 0; 0 0 1]
  Rigid Transform6 : sm_lib/Frames and Transforms/Rigid Transform  TranslationMethod=Cartesian  TranslationStandardOffset=0.3  TranslationLengthUnit=mm  TranslationStandardAxis=+X  TranslationCartesianOffset=Hip.legGbxOft  TranslationROffset=0  TranslationROffsetUnits=m  TranslationZOffset=0  TranslationZOffsetUnits=m  TranslationThetaOffset=0  TranslationThetaOffsetUnits=deg  RotationMethod=StandardAxis  RotationAngleUnits=deg  RotationStandardAxis=-X  RotationAngle=90  RotationArbitraryAxis=[0 0 1]  FollAlignAxisA=+X  BaseAlignAxisA=+Y  FollAlignAxisB=+Y  BaseAlignAxisB=+Z  RotationSequenceAxes=FollowerAxes  RotationSequence=XYX  RotationSequenceAngles=[0 0 0]  RotationSequenceAnglesUnits=deg  RotationMatrix=[1 0 0; 0 1 0; 0 0 1]
  Rigid Transform7 : sm_lib/Frames and Transforms/Rigid Transform  TranslationMethod=Cartesian  TranslationStandardOffset=0.3  TranslationLengthUnit=mm  TranslationStandardAxis=+X  TranslationCartesianOffset=Hip.legOft  TranslationROffset=0  TranslationROffsetUnits=m  TranslationZOffset=0  TranslationZOffsetUnits=m  TranslationThetaOffset=0  TranslationThetaOffsetUnits=deg  RotationMethod=RotationSequence  RotationAngleUnits=deg  RotationStandardAxis=-X  RotationAngle=180  RotationArbitraryAxis=[0 0 1]  FollAlignAxisA=+X  BaseAlignAxisA=+Y  FollAlignAxisB=+Y  BaseAlignAxisB=+Z  RotationSequenceAxes=FollowerAxes  RotationSequence=XYZ  RotationSequenceAngles=[0 0 180]  RotationSequenceAnglesUnits=deg  RotationMatrix=[1 0 0; 0 1 0; 0 0 1]
  Rigid Transform8 : sm_lib/Frames and Transforms/Rigid Transform  TranslationMethod=Cartesian  TranslationStandardOffset=0.3  TranslationLengthUnit=mm  TranslationStandardAxis=+X  TranslationCartesianOffset=Hip.kneeGbxOft  TranslationROffset=0  TranslationROffsetUnits=m  TranslationZOffset=0  TranslationZOffsetUnits=m  TranslationThetaOffset=0  TranslationThetaOffsetUnits=deg  RotationMethod=StandardAxis  RotationAngleUnits=deg  RotationStandardAxis=-X  RotationAngle=90  RotationArbitraryAxis=[0 0 1]  FollAlignAxisA=+X  BaseAlignAxisA=+Y  FollAlignAxisB=+Y  BaseAlignAxisB=+Z  RotationSequenceAxes=FollowerAxes  RotationSequence=XYX  RotationSequenceAngles=[0 0 0]  RotationSequenceAnglesUnits=deg  RotationMatrix=[1 0 0; 0 1 0; 0 0 1]
  Spatial Contact Force : sm_lib/Forces and Torques/Spatial Contact Force  CoefficientOfDynamicFriction=Hip.kine_frict  CoefficientOfStaticFriction=Hip.stat_frict  NormalDamping=1e3  NormalDampingUnits=N/(m/s)  NormalStiffness=1e6  NormalStiffnessUnits=N/m  FrictionalCriticalVelocity=1e-3  FrictionalCriticalVelocityUnits=m/s  SenseFrictionalForceMagnitude=off  SenseNormalForceMagnitude=on  SenseSeparationDistance=off  NormalTransitionRegionWidth=1e-4  NormalTransitionRegionWidthUnits=m  FrictionType=SmoothStickSlip
      settings: SourceProductName=Simscape Multibody
  Spherical Solid : sm_lib/Body Elements/Spherical Solid  GraphicAmbientColor=[0.15 0.15 0.15 1.0]  BasedOnType=Density  CenterOfMass=[0 0 0]  CenterOfMassUnits=m  GraphicDiffuseColor=[1.0 1.0 1.0]  Density=1000  DensityUnits=kg/m^3  DoExposeReferenceFrame=on  GraphicEmissiveColor=[0.0 0.0 0.0 1.0]  ExportEntireGeometry=on  SerializedExposedGeometries=<ExposedGeometries><ExposedGeometry><RawGeometryId>entire</RawGeometryId><ExposedGeometryId>G</ExposedGeometryId></ExposedGeometry></ExposedGeometries>  SerializedFrames=<Frames/>  MarkerShape=Sphere  MarkerSize=10  GraphicType=FromGeometry  InertiaType=CalculateFromGeometry  Mass=1  MassUnits=kg  MomentsOfInertia=[1 1 1]  MomentsOfInertiaUnits=kg*m^2  GraphicOpacity=0.05  ProductsOfInertia=[0 0 0]  ProductsOfInertiaUnits=kg*m^2  GraphicShininess=75  GraphicSpecularColor=[0.5 0.5 0.5 1.0]  SphereRadius=Hip.sphere_rad  SphereRadiusUnits=m  GraphicVisPropType=SimpleVisualProperties
      settings: SourceProductName=Simscape Multibody
  hip motor : sm_lib/Body Elements/Cylindrical Solid  GraphicAmbientColor=[0.15 0.15 0.15 1.0]  BasedOnType=Mass  CenterOfMass=[0 0 0]  CenterOfMassUnits=m  GraphicDiffuseColor=Hip.GbxColor  CylinderLength=Hip.gearboxThickness  CylinderLengthUnits=mm  CylinderRadius=Hip.gearboxRadius  CylinderRadiusUnits=mm  Density=1000  DensityUnits=kg/m^3  DoExposeReferenceFrame=on  GraphicEmissiveColor=[0.0 0.0 0.0 1.0]  ExportEntireGeometry=off  SerializedFrames=<Frames/>  MarkerShape=Sphere  MarkerSize=10  GraphicType=FromGeometry  InertiaType=CalculateFromGeometry  Mass=Hip.gearboxMass  MassUnits=g  MomentsOfInertia=[1 1 1]  MomentsOfInertiaUnits=kg*m^2  GraphicOpacity=1.0  ProductsOfInertia=[0 0 0]  ProductsOfInertiaUnits=kg*m^2  GraphicShininess=75  GraphicSpecularColor=[0.5 0.5 0.5 1.0]  GraphicVisPropType=SimpleVisualProperties
  joint : Subsystem  mask{Joint=Hip.joint}
  knee motor : sm_lib/Body Elements/Cylindrical Solid  GraphicAmbientColor=[0.15 0.15 0.15 1.0]  BasedOnType=Mass  CenterOfMass=[0 0 0]  CenterOfMassUnits=m  GraphicDiffuseColor=Hip.GbxColor  CylinderLength=Hip.gearboxThickness  CylinderLengthUnits=mm  CylinderRadius=Hip.gearboxRadius  CylinderRadiusUnits=mm  Density=1000  DensityUnits=kg/m^3  DoExposeReferenceFrame=on  GraphicEmissiveColor=[0.0 0.0 0.0 1.0]  ExportEntireGeometry=off  SerializedFrames=<Frames/>  MarkerShape=Sphere  MarkerSize=10  GraphicType=FromGeometry  InertiaType=CalculateFromGeometry  Mass=Hip.gearboxMass  MassUnits=g  MomentsOfInertia=[1 1 1]  MomentsOfInertiaUnits=kg*m^2  GraphicOpacity=1.0  ProductsOfInertia=[0 0 0]  ProductsOfInertiaUnits=kg*m^2  GraphicShininess=75  GraphicSpecularColor=[0.5 0.5 0.5 1.0]  GraphicVisPropType=SimpleVisualProperties
  leg motor : sm_lib/Body Elements/Cylindrical Solid  GraphicAmbientColor=[0.15 0.15 0.15 1.0]  BasedOnType=Mass  CenterOfMass=[0 0 0]  CenterOfMassUnits=m  GraphicDiffuseColor=Hip.GbxColor  CylinderLength=Hip.gearboxThickness  CylinderLengthUnits=mm  CylinderRadius=Hip.gearboxRadius  CylinderRadiusUnits=mm  Density=1000  DensityUnits=kg/m^3  DoExposeReferenceFrame=on  GraphicEmissiveColor=[0.0 0.0 0.0 1.0]  ExportEntireGeometry=off  SerializedFrames=<Frames/>  MarkerShape=Sphere  MarkerSize=10  GraphicType=FromGeometry  InertiaType=CalculateFromGeometry  Mass=Hip.gearboxMass  MassUnits=g  MomentsOfInertia=[1 1 1]  MomentsOfInertiaUnits=kg*m^2  GraphicOpacity=1.0  ProductsOfInertia=[0 0 0]  ProductsOfInertiaUnits=kg*m^2  GraphicShininess=75  GraphicSpecularColor=[0.5 0.5 0.5 1.0]  GraphicVisPropType=SimpleVisualProperties
  B : PMIOPort  Side=Left
  F : PMIOPort  Port=2  Side=Right
  plane : PMIOPort  Port=3  Side=Right
  p : Outport
  wires:
  pos/1 -> joint/1(in)
  joint/1(p) -> Bus Creator/1  "joint"
  PS-Simulink Converter/1 -> Bus Creator/2  "normal_force"
  Bus Creator/1 -> p/1
  connections:
  Rigid Transform7/RConn1 -- F/RConn1
  Rigid Transform6/RConn1 -- leg motor/RConn1 -- Rigid Transform7/LConn1
  Rigid Transform8/RConn1 -- knee motor/RConn1 -- Spherical Solid/RConn1
  B/RConn1 -- Rigid Transform1/LConn1
  Rigid Transform6/LConn1 -- Rigid Transform8/LConn1 -- joint/RConn1 -- hip motor/RConn1
  Rigid Transform1/RConn1 -- joint/LConn1
  Spatial Contact Force/LConn1 -- Spherical Solid/LConn1
  plane/RConn1 -- Spatial Contact Force/RConn1
  Spatial Contact Force/RConn2 -- PS-Simulink Converter/LConn1
